simulink model "Hinf_Simulink"  (R2019b)
settings: Solver=ode15s  StartTime=0.0  StopTime=20  RelTol=1e-3
values from neighbouring files (symbols this model uses):
  Co = [1 0 0 0; 0 0 1 0]    [Hinf_Controlled.m]
  X0 = [0,0,pi*15/16,0]'    [Hinf_Controlled.m]
undefined symbols (not defined in the file or in its folder): K
settings Model: Creator=000  LastModifiedBy=000

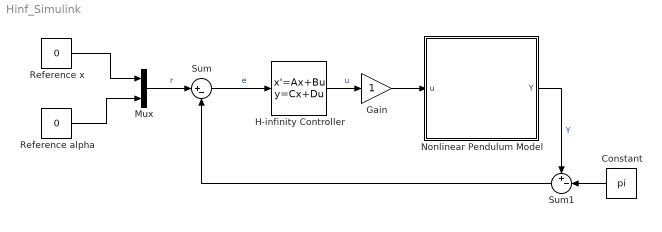
== system Hinf_Simulink ==
  Constant : Constant  Value=pi
  Gain : Gain
  H-infinity Controller : StateSpace  A=K.A  B=K.B  C=K.C  D=K.D  InitialCondition=0
  Mux : Mux  Inputs=2
  Nonlinear Pendulum Model : Subsystem
  Reference alpha : Constant  Value=0
  Reference x : Constant  Value=0
  Sum : Sum  Inputs=|+-
  Sum1 : Sum  Inputs=+-|
  wires:
  Nonlinear Pendulum Model/1(Y) -> Sum1/1  "Y"
  Sum/1 -> H-infinity Controller/1  "e"
  Mux/1 -> Sum/1  "r"
  Reference x/1 -> Mux/1
  Reference alpha/1 -> Mux/2
  H-infinity Controller/1 -> Gain/1  "u"
  Gain/1 -> Nonlinear Pendulum Model/1(u)
  Sum1/1 -> Sum/2
  Constant/1 -> Sum1/2

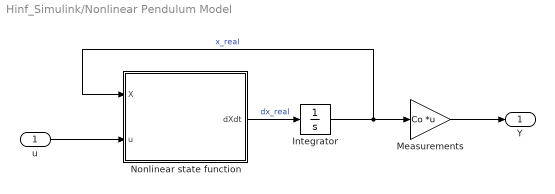
== system Hinf_Simulink/Nonlinear Pendulum Model ==
  u : Inport
  Integrator : Integrator  InitialCondition=X0
  Measurements : Gain  Gain=Co  Multiplication=Matrix(K*u)
  "Nonlinear state function " : MATLAB Function  TreatAsAtomicUnit=on
  Y : Outport
  wires:
  "Nonlinear state function "/1(dXdt) -> Integrator/1  "dx_real"
  u/1 -> "Nonlinear state function "/2(u)
  Integrator/1 -> Measurements/1, "Nonlinear state function "/1(X)  "x_real"
  Measurements/1 -> Y/1

== matlab function Hinf_Simulink/Nonlinear Pendulum Model/Nonlinear state function  ==
  data: X input; u input; dXdt output
function dXdt = pendCartC(X,u)
%PENDCARTC
%    DXDT = PENDCARTC(IN1,U)

%    This function was generated by the Symbolic Math Toolbox version 8.4.
%    19-May-2020 20:15:22

X2 = X(2,:);
X3 = X(3,:);
X4 = X(4,:);
t2 = cos(X3);
t3 = sin(X3);
t4 = X4.^2;
t5 = t2.^2;
t6 = t5.*4.565807400625001e-4;
t7 = t6-3.005650706948956e-3;
t8 = 1.0./t7;
dXdt = [X2;t8.*(X2.*(-5.665253057117538e-6)+u.*5.387661376655595e-7+X4.*t2.*5.3763908601e-9+t2.*t3.*4.695776235861861e-7+t3.*t4.*1.074185854609239e-8).*(-9.53848061542277e+3);X4;t8.*(X4.*1.57714169184e-7+t3.*1.377486248645154e-5-X2.*t2.*2.524516833955624e-5+t2.*u.*2.40081805770912e-6+t2.*t3.*t4.*4.786723991704242e-8).*9.53848061542277e+3];
